simulink library "mtq_model_lib"  (R2018b)
settings: Solver=VariableStepAuto  StartTime=0.0  StopTime=10.0  RelTol=1e-3
libraries: powerlib_meascontrol x1
settings Model: Creator=taylorreynolds  LastModifiedBy=taylorreynolds

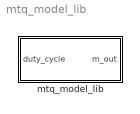
== system mtq_model_lib ==
  mtq_model_lib : Subsystem  mask{R=23.2, L=0.2, Vs=5, Fsw=10000, NA=0.23896}
      mask prompts: R "Track Resistance [Ohms]"; L "Track Inductance [Henry]"; Vs "Driving voltage [V]"; Fsw "PWM frequency [Hz]"; NA "Product of # turns and enclosed area (N x A)"
      mask TypeOptions R: R/Gain
      mask TypeOptions L: L/Value
      mask TypeOptions Vs: Vs/Gain
      mask TypeOptions Fsw:
      | PWM Generator
      | (DC-DC)/Fsw
      mask TypeOptions NA: NA/Gain
      mask DialogControl DescGroupVar Prompt: AACT GNC Simulation Tool
      mask DialogControl DescTextVar Prompt: SOC-i magnetorquer model

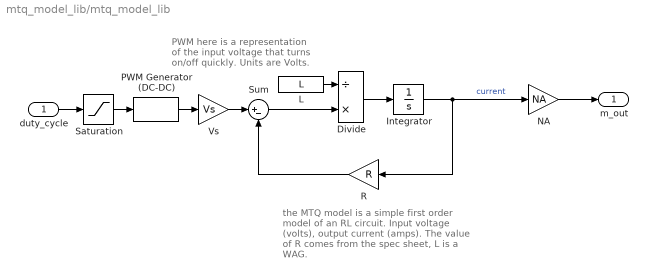
== system mtq_model_lib/mtq_model_lib ==
  note: PWM here is a representation of the input voltage
      | that turns on/off quickly. Units are Volts.
  note: the MTQ model is a simple first order model of an RL circuit. Input voltage (volts), output current (amps).
      | The value of R comes from the spec sheet, L is a WAG.
  duty_cycle : Inport
  Divide : Product  Inputs=/*
  Integrator : Integrator
  L : Constant  Value=L
  NA : Gain  Gain=NA
  PWM Generator (DC-DC) : powerlib_meascontrol/Pulse & Signal Generators/PWM Generator (DC-DC)  Fsw=Fsw  Ts=0
  R : Gain  Gain=R
  Saturation : Saturate  UpperLimit=1  LowerLimit=0  LinearizeAsGain=off
  Sum : Sum  Inputs=|+-
  Vs : Gain  Gain=Vs
  m_out : Outport
  wires:
  PWM Generator (DC-DC)/1 -> Vs/1
  Vs/1 -> Sum/1
  Saturation/1 -> PWM Generator (DC-DC)/1
  L/1 -> Divide/1
  Divide/1 -> Integrator/1
  Sum/1 -> Divide/2
  R/1 -> Sum/2
  NA/1 -> m_out/1
  Integrator/1 -> NA/1, R/1  "current"
  duty_cycle/1 -> Saturation/1
